simulink model "BatteryModelLUTtotal2RC"  (R2019a)
settings: Solver=VariableStepAuto  StartTime=0.0  StopTime=2417.4  RelTol=1e-3
undefined symbols (not defined in the file): Ah, C1new, C2new, DiscIntNeverNeededParam, Emnew, Idis, R0new, R1new, R2new, SOCnew
settings Model: Creator=danis  LastModifiedBy=danis

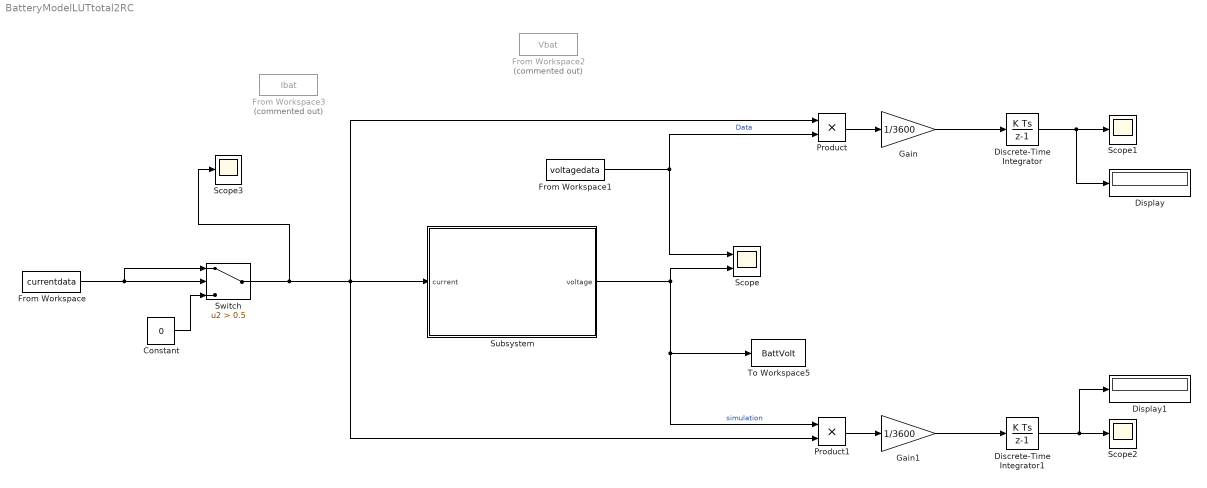
== system BatteryModelLUTtotal2RC ==
  Constant : Constant  Value=0
  Discrete-Time Integrator : DiscreteIntegrator  SampleTime=-1  ICPrevOutput=DiscIntNeverNeededParam  ICPrevScaledInput=DiscIntNeverNeededParam
  Discrete-Time Integrator1 : DiscreteIntegrator  SampleTime=-1  ICPrevOutput=DiscIntNeverNeededParam  ICPrevScaledInput=DiscIntNeverNeededParam
  Display : Display
  Display1 : Display
  From Workspace : FromWorkspace  VariableName=currentdata  SampleTime=0.001
  From Workspace1 : FromWorkspace  VariableName=voltagedata  SampleTime=0.001
  From Workspace2 : FromWorkspace  Commented=on  VariableName=Vbat  SampleTime=0.001  Interpolate=off  OutputAfterFinalValue=Cyclic repetition
  From Workspace3 : FromWorkspace  Commented=on  VariableName=Ibat  SampleTime=0.001  Interpolate=off  OutputAfterFinalValue=Cyclic repetition
  Gain : Gain  Gain=1/3600
  Gain1 : Gain  Gain=1/3600
  Product : Product
  Product1 : Product
  Scope : Scope  NumInputPorts=2
  Scope1 : Scope
  Scope2 : Scope
  Scope3 : Scope
  Subsystem : Subsystem
  Switch : Switch  Criteria=u2 > Threshold  Threshold=0.5
  To Workspace5 : ToWorkspace  VariableName=BattVolt  SampleTime=-1
  wires:
  From Workspace1/1 -> Scope/1, Product/2  "Data"
  Subsystem/1(voltage) -> Product1/1, To Workspace5/1, Scope/2  "simulation"
  Product/1 -> Gain/1
  Gain/1 -> Discrete-Time Integrator/1
  Discrete-Time Integrator/1 -> Display/1, Scope1/1
  Discrete-Time Integrator1/1 -> Display1/1, Scope2/1
  Gain1/1 -> Discrete-Time Integrator1/1
  Product1/1 -> Gain1/1
  From Workspace/1 -> Switch/1, Switch/2
  Switch/1 -> Scope3/1, Product1/2, Product/1, Subsystem/1(current)
  Constant/1 -> Switch/3

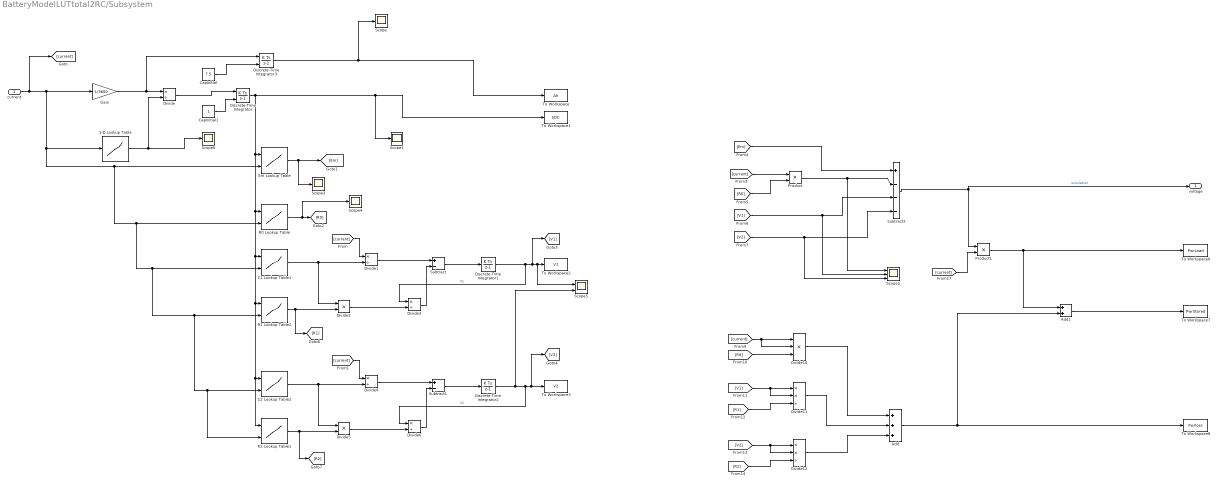
== system BatteryModelLUTtotal2RC/Subsystem ==
  current : Inport
  1-D Lookup Table : Lookup_n-D  NumberOfTableDimensions=1  BreakpointsForDimension1=Idis  Table=Ah  InternalRulePriority=Speed  RndMeth=Simplest  InputSameDT=on
  Add : Sum  Inputs=+++
  Add1 : Sum
  C1 Lookup Table1 : Lookup_n-D  BreakpointsForDimension1=SOCnew  BreakpointsForDimension2=Idis  Table=C1new  InternalRulePriority=Speed  RndMeth=Simplest  InputSameDT=on
  C2 Lookup Table2 : Lookup_n-D  BreakpointsForDimension1=SOCnew  BreakpointsForDimension2=Idis  Table=C2new  InternalRulePriority=Speed  RndMeth=Simplest  InputSameDT=on
  CapInitial : Constant  Value=7.5  SampleTime=0.001
  CapInitial1 : Constant  SampleTime=0.001
  Discrete-Time Integrator : DiscreteIntegrator  InitialConditionSource=external  SampleTime=-1  ICPrevOutput=DiscIntNeverNeededParam  ICPrevScaledInput=DiscIntNeverNeededParam
  Discrete-Time Integrator1 : DiscreteIntegrator  SampleTime=-1  ICPrevOutput=DiscIntNeverNeededParam  ICPrevScaledInput=DiscIntNeverNeededParam
  Discrete-Time Integrator2 : DiscreteIntegrator  SampleTime=-1  ICPrevOutput=DiscIntNeverNeededParam  ICPrevScaledInput=DiscIntNeverNeededParam
  Discrete-Time Integrator3 : DiscreteIntegrator  InitialConditionSource=external  SampleTime=-1  ICPrevOutput=DiscIntNeverNeededParam  ICPrevScaledInput=DiscIntNeverNeededParam
  Divide{,1,3..4,6} (5 alike) : Product  Inputs=*/
  Divide10 : Product  Inputs=***
  Divide11 : Product  Inputs=**/
  Divide12 : Product  Inputs=**/
  Divide2 : Product  Inputs=**
  Divide5 : Product  Inputs=**
  Em Lookup Table : Lookup_n-D  BreakpointsForDimension1=SOCnew  BreakpointsForDimension2=Idis  Table=Emnew  InternalRulePriority=Speed  RndMeth=Simplest  InputSameDT=on
  Gain : Gain  Gain=-1/3600
  Product : Product
  Product1 : Product
  R0 Lookup Table : Lookup_n-D  BreakpointsForDimension1=SOCnew  BreakpointsForDimension2=Idis  Table=R0new  InternalRulePriority=Speed  RndMeth=Simplest  InputSameDT=on
  R1 Lookup Table2 : Lookup_n-D  BreakpointsForDimension1=SOCnew  BreakpointsForDimension2=Idis  Table=R1new  InternalRulePriority=Speed  RndMeth=Simplest  InputSameDT=on
  R2 Lookup Table1 : Lookup_n-D  BreakpointsForDimension1=SOCnew  BreakpointsForDimension2=Idis  Table=R2new  InternalRulePriority=Speed  RndMeth=Simplest  InputSameDT=on
  Scope{,1,3..4,6} (5 alike) : Scope
  Scope2 : Scope  NumInputPorts=3
  Scope5 : Scope  NumInputPorts=2
  Subtract : Sum  Inputs=+-
  Subtract1 : Sum  Inputs=+-
  Subtract3 : Sum  Inputs=+---
  To Workspace : ToWorkspace  VariableName=Ah  SampleTime=-1
  To Workspace1 : ToWorkspace  VariableName=SOC  SampleTime=-1
  To Workspace2 : ToWorkspace  VariableName=V1  SampleTime=-1
  To Workspace3 : ToWorkspace  VariableName=V2  SampleTime=-1
  To Workspace6 : ToWorkspace  VariableName=PwrLoad  SampleTime=-1
  To Workspace7 : ToWorkspace  VariableName=PwrStored  SampleTime=-1
  To Workspace8 : ToWorkspace  VariableName=Pwrloss  SampleTime=-1
  voltage : Outport
  wires:
  Discrete-Time Integrator2/1 -> Scope5/2, Divide6/1, To Workspace3/1, [V2]  "V2"
  Divide4/1 -> Subtract1/1
  [R0] -> Product/2
  C2 Lookup Table2/1 -> Divide5/1, Divide4/2
  C1 Lookup Table1/1 -> Divide2/1, Divide1/2
  [current] -> Product1/2
  Divide3/1 -> Subtract/2
  Divide6/1 -> Subtract1/2
  [Em] -> Subtract3/1
  Divide5/1 -> Divide6/2
  Subtract/1 -> Discrete-Time Integrator1/1
  R2 Lookup Table1/1 -> [R2], Divide5/2
  Divide2/1 -> Divide3/2
  Divide1/1 -> Subtract/1
  1-D Lookup Table/1 -> Divide/2, Scope6/1
  [current] -> Divide10/2, Divide10/1
  Discrete-Time Integrator1/1 -> Divide3/1, Scope5/1, To Workspace2/1, [V1]  "V1"
  Divide10/1 -> Add/1
  [V1] -> Divide11/2, Divide11/1
  Subtract1/1 -> Discrete-Time Integrator2/1
  [current] -> Product/1
  [current] -> Divide4/1
  [V2] -> Scope2/3, Subtract3/4
  [R1] -> Divide11/3
  R1 Lookup Table2/1 -> [R1], Divide2/2
  Product/1 -> Scope2/1, Subtract3/2
  Em Lookup Table/1 -> Scope3/1, [Em]
  [V1] -> Scope2/2, Subtract3/3
  [R0] -> Divide10/3
  Divide11/1 -> Add/2
  [current] -> Divide1/1
  Divide12/1 -> Add/3
  R0 Lookup Table/1 -> Scope4/1, [R0]
  [R2] -> Divide12/3
  Subtract3/1 -> voltage/1, Product1/1  "simulation"
  Add1/1 -> To Workspace7/1
  [V2] -> Divide12/2, Divide12/1
  Add/1 -> To Workspace8/1, Add1/2
  Product1/1 -> To Workspace6/1, Add1/1
  current/1 -> [current], R2 Lookup Table1/2, C2 Lookup Table2/2, R1 Lookup Table2/2, C1 Lookup Table1/2, R0 Lookup Table/2, Em Lookup Table/2, 1-D Lookup Table/1, Gain/1
  Divide/1 -> Discrete-Time Integrator/1
  CapInitial/1 -> Discrete-Time Integrator3/2
  Discrete-Time Integrator/1 -> Em Lookup Table/1, R2 Lookup Table1/1, C2 Lookup Table2/1, R1 Lookup Table2/1, C1 Lookup Table1/1, R0 Lookup Table/1, Scope1/1, To Workspace1/1
  Gain/1 -> Discrete-Time Integrator3/1, Divide/1
  Discrete-Time Integrator3/1 -> Scope/1, To Workspace/1
  CapInitial1/1 -> Discrete-Time Integrator/2
